simulink model "ap4"  (Simulink 7.1)
settings: Solver=ode45  StartTime=0.0  StopTime=10.0  RelTol=1e-3
settings Model: Creator=madalin  LastModifiedBy=madalin

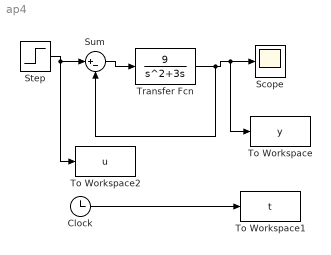
== system ap4 ==
  Clock : Clock
      settings: Decimation=10
  Scope : Scope
  Step : Step  SampleTime=0
  Sum : Sum  Inputs=|+-  OutDataType=sfix(16)  OutScaling=2^0
  To Workspace : ToWorkspace  VariableName=y  SampleTime=-1  SaveFormat=Array
  To Workspace1 : ToWorkspace  VariableName=t  SampleTime=-1  SaveFormat=Array
  To Workspace2 : ToWorkspace  VariableName=u  SampleTime=-1  SaveFormat=Structure
  Transfer Fcn : TransferFcn  Numerator=[9]  Denominator=[1 3 0]
  wires:
  Step/1 -> Sum/1, To Workspace2/1
  Sum/1 -> Transfer Fcn/1
  Transfer Fcn/1 -> Sum/2, Scope/1, To Workspace/1
  Clock/1 -> To Workspace1/1
